simulink library "fixed_ground_station_ul"  (R2018b)
settings: Solver=VariableStepAuto  StartTime=0.0  StopTime=10.0  RelTol=1e-3
values from neighbouring files (symbols this model uses):
  c_damp = 0.5    [fixed_ground_station_ts.m]
  Izz = 1    [fixed_ground_station_ts.m]
undefined symbols (not defined in the file or in its folder): class_thr, ini_OwP, ini_psiPlat
libraries: calcTetherEndNodesStates x1, sumTetherForcesAndMoments_ul x1
settings Model: Creator=Ayaz  LastModifiedBy=Ayaz

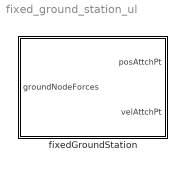
== system fixed_ground_station_ul ==
  fixedGroundStation : Subsystem  mask{Izz=Izz, plat_damp_coeff=c_damp, thr_struct=class_thr}
      mask prompts: Izz "Moment of inertia about Z"; plat_damp_coeff "Damping Coefficient"; thr_struct "Tether field"
      mask TypeOptions thr_struct: sumTetherForcesAndMoments/thr_struct
      mask DialogControl Ground_station Prompt: Ground Station Variables
      mask DialogControl Tether Prompt: Tether Variable

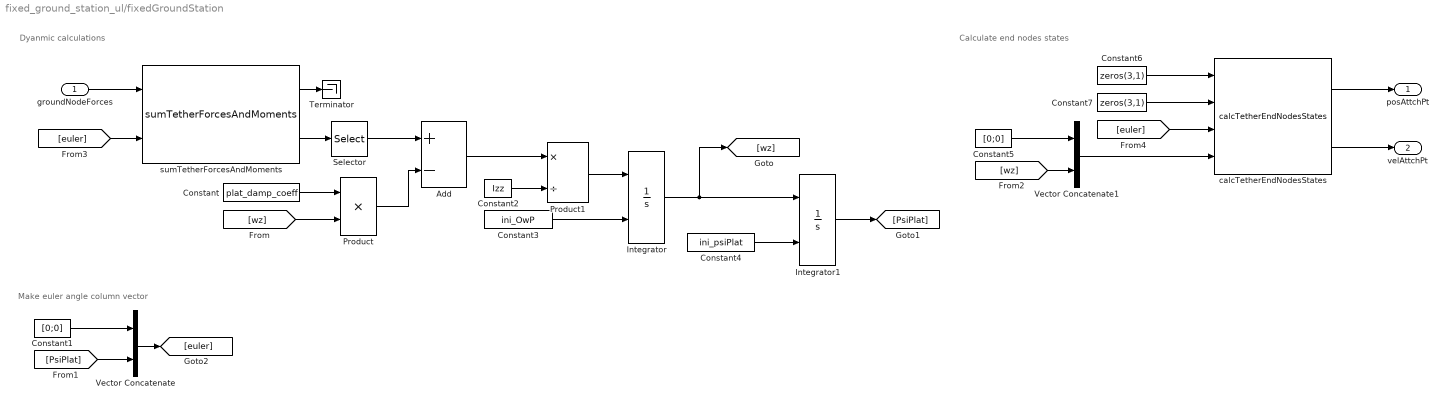
== system fixed_ground_station_ul/fixedGroundStation ==
  note: Dyanmic calculations
  note: Make euler angle column vector
  note: Calculate end nodes states
  groundNodeForces : Inport
  Add : Sum  Inputs=+-
  Constant : Constant  Value=plat_damp_coeff  VectorParams1D=off
  Constant1 : Constant  Value=[0;0]  VectorParams1D=off
  Constant2 : Constant  Value=Izz  VectorParams1D=off
  Constant3 : Constant  Value=ini_OwP  VectorParams1D=off
  Constant4 : Constant  Value=ini_psiPlat  VectorParams1D=off
  Constant5 : Constant  Value=[0;0]  VectorParams1D=off
  Constant6 : Constant  Value=zeros(3,1)  VectorParams1D=off
  Constant7 : Constant  Value=zeros(3,1)  VectorParams1D=off
  Integrator : Integrator  InitialConditionSource=external
  Integrator1 : Integrator  InitialConditionSource=external
  Product : Product
  Product1 : Product  Inputs=*/
  Selector : Selector  InputPortWidth=3  IndexOptions=Index vector (dialog)  Indices=3  OutputSizes=1
  Terminator : Terminator
  Vector Concatenate : Concatenate
  Vector Concatenate1 : Concatenate
  calcTetherEndNodesStates : calcTetherEndNodesStates/calcTetherEndNodesStates  thr_struct=class_thr  attach_point=Ground station
  sumTetherForcesAndMoments : sumTetherForcesAndMoments_ul/sumTetherForcesAndMoments  thr_struct=thr_struct  attach_point=Ground station
  posAttchPt : Outport
  velAttchPt : Outport  Port=2
  wires:
  groundNodeForces/1 -> sumTetherForcesAndMoments/1
  sumTetherForcesAndMoments/1 -> Terminator/1
  sumTetherForcesAndMoments/2 -> Selector/1
  Selector/1 -> Add/1
  Constant/1 -> Product/1
  [wz] -> Product/2
  Product/1 -> Add/2
  Add/1 -> Product1/1
  Constant2/1 -> Product1/2
  Product1/1 -> Integrator/1
  Constant3/1 -> Integrator/2
  Integrator/1 -> Integrator1/1, [wz]
  Integrator1/1 -> [PsiPlat]
  Constant4/1 -> Integrator1/2
  [PsiPlat] -> Vector Concatenate/2
  Constant1/1 -> Vector Concatenate/1
  Constant5/1 -> Vector Concatenate1/1
  [wz] -> Vector Concatenate1/2
  Vector Concatenate1/1 -> calcTetherEndNodesStates/4
  Vector Concatenate/1 -> [euler]
  [euler] -> sumTetherForcesAndMoments/2
  [euler] -> calcTetherEndNodesStates/3
  Constant7/1 -> calcTetherEndNodesStates/2
  Constant6/1 -> calcTetherEndNodesStates/1
  calcTetherEndNodesStates/2 -> velAttchPt/1
  calcTetherEndNodesStates/1 -> posAttchPt/1
